simulink model "mpcModel"  (R2020a)
settings: Solver=FixedStepAuto  StartTime=0.0  StopTime=MPCSim_path.Duration  FixedStep=MPCSim_path.Ts  RelTol=1e-3
values from neighbouring files (symbols this model uses):
  PosXY = [0,x(2)]    [run_MPCPath.m]
  x = xHistory(k,:)    [run_MPCPath.m]
undefined symbols (not defined in the file or in its folder): MPCParam_path, MPCSim_path
libraries: simulink x1
settings Model: Creator=sl  LastModifiedBy=sl

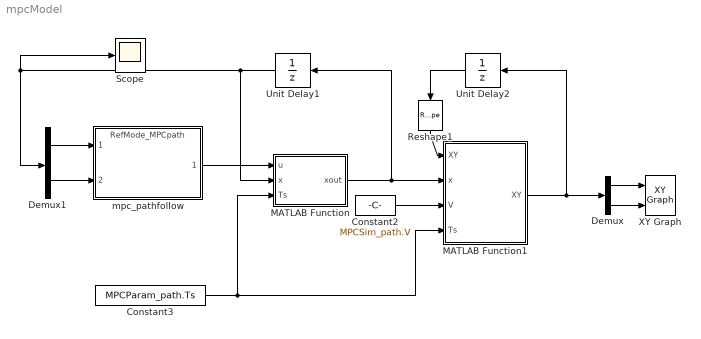
== system mpcModel ==
  Constant2 : Constant  Value=MPCSim_path.V
  Constant3 : Constant  Value=MPCParam_path.Ts
  Demux : Demux  Outputs=2
  Demux1 : Demux  Outputs=2
  MATLAB Function : MATLAB Function  TreatAsAtomicUnit=on
  MATLAB Function1 : MATLAB Function  TreatAsAtomicUnit=on
  Reshape1 : Reshape  OutputDimensionality=Customize  OutputDimensions=[1,2]
  Scope : Scope
  Unit Delay1 : UnitDelay  InitialCondition=x  SampleTime=-1  HasFrameUpgradeWarning=on
  Unit Delay2 : UnitDelay  InitialCondition=PosXY(1,:)  SampleTime=-1  HasFrameUpgradeWarning=on
  XY Graph : simulink/Sinks/XY Graph  xmin=-100  xmax=200  ymin=-100  ymax=100  st=-1
  mpc_pathfollow : ModelReference  ModelNameDialog=RefMode_MPCpath  SimulationMode=Normal  ModelReferenceVersion=1.56
  wires:
  MATLAB Function/1(xout) -> Unit Delay1/1, MATLAB Function1/2(x)
  Unit Delay1/1 -> Demux1/1, Scope/1, MATLAB Function/2(x)
  MATLAB Function1/1(XY) -> Demux/1, Unit Delay2/1
  Unit Delay2/1 -> Reshape1/1
  Constant2/1 -> MATLAB Function1/3(V)
  Constant3/1 -> MATLAB Function/3(Ts), MATLAB Function1/4(Ts)
  Reshape1/1 -> MATLAB Function1/1("XY ")
  Demux/1 -> XY Graph/1
  Demux/2 -> XY Graph/2
  mpc_pathfollow/1 -> MATLAB Function/1(u)
  Demux1/1 -> mpc_pathfollow/1
  Demux1/2 -> mpc_pathfollow/2

== matlab function mpcModel/MATLAB Function1 ==
  data: XY input; x input; XY output; V input; Ts input
function XY= fcn(XY, x, V, Ts)
XY = XY + V*[cos(x(1)) sin(x(1))]*Ts;

== matlab function mpcModel/MATLAB Function ==
  data: u input; xout output; x input; Ts input
function xout = fcn(u,x,Ts)
xout = x+uavPathFollowStateFcn(x,u)*Ts;
